simulink model "P1"  (R2020a)
settings: Solver=VariableStepAuto  StartTime=0  StopTime=10.0  RelTol=1e-3
settings Model: Creator=Jason  LastModifiedBy=Jason

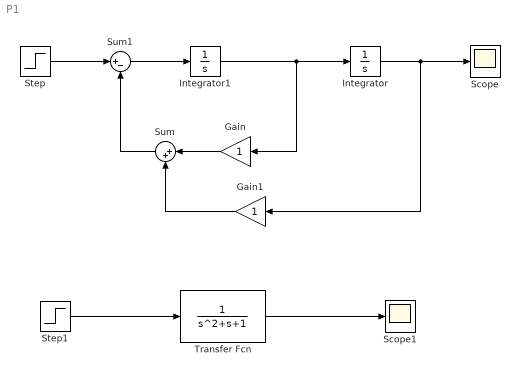
== system P1 ==
  Gain : Gain
  Gain1 : Gain
  Integrator : Integrator
  Integrator1 : Integrator
  Scope : Scope
  Scope1 : Scope
  Step : Step  SampleTime=0
  Step1 : Step  SampleTime=0
  Sum : Sum  Inputs=|++
  Sum1 : Sum  Inputs=|+-
  Transfer Fcn : TransferFcn  Denominator=[1 1 1]
  wires:
  Sum1/1 -> Integrator1/1
  Integrator1/1 -> Gain/1, Integrator/1
  Gain1/1 -> Sum/2
  Gain/1 -> Sum/1
  Integrator/1 -> Gain1/1, Scope/1
  Sum/1 -> Sum1/2
  Step/1 -> Sum1/1
  Step1/1 -> Transfer Fcn/1
  Transfer Fcn/1 -> Scope1/1
